simulink model "backlash_like"  (R2025b)
settings: Solver=VariableStepAuto  StartTime=0.0  StopTime=0.02  MaxStep=1e-5  RelTol=1e-3
settings Model: Creator=user  LastModifiedBy=PME406_01
settings SolverCC: AlgebraicLoopSolver=TrustRegion
settings DataIOCC: ReturnWorkspaceOutputs=off
settings DebuggingCC: UnconnectedInputMsg=warning  UnconnectedOutputMsg=warning  UnconnectedLineMsg=warning  ArithmeticOperatorsInVariantConditions=warning
settings ModelReferenceCC: EnableRefExpFcnMdlSchedulingChecks=on
settings SFSimCC: SimUseLocalCustomCode=off  CustomCodeUndefinedFunction=UseInterfaceOnly
settings RTWCC: RTWUseLocalCustomCode=off  GPUComputeCapability=3.5
settings CodeAppCC: StateflowObjectComments=on

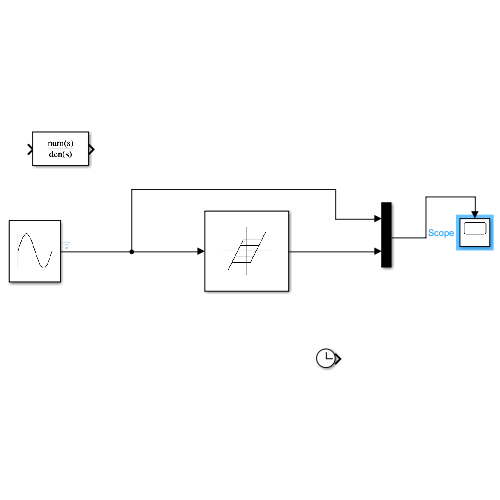
[thumbnail: Simulink's stored preview of the top-level diagram]
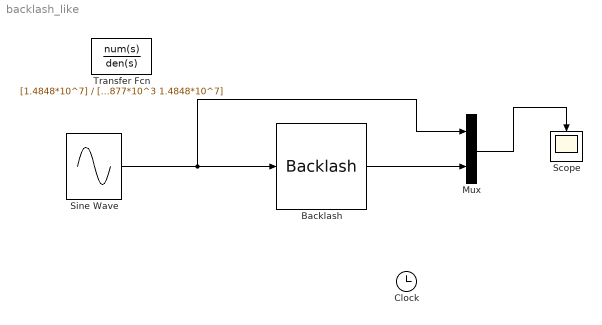
== system backlash_like ==
  Backlash : Backlash  BacklashWidth=0.01
  Clock : Clock
  Mux : Mux  Inputs=2
  Scope : Scope
      settings: ActiveDisplayYMinimum=-0.91147137767863  ActiveDisplayYMaximum=-0.8543896051558113
  Sine Wave : Sin  Bias=0.1  Frequency=2*pi*100
  Transfer Fcn : TransferFcn  Numerator=[1.4848*10^7]  Denominator=[1 8.1877*10^3 1.4848*10^7]
  wires:
  Backlash/1 -> Mux/2
  Mux/1 -> Scope/1
  Sine Wave/1 -> Mux/1, Backlash/1
